simulink model "sampleModel1609"  (R2023a)
settings: Solver=VariableStepAuto  StartTime=0.0  StopTime=10.0  RelTol=1e-3
libraries: hdlsllib x6
settings Model: Creator=user1  LastModifiedBy=user1

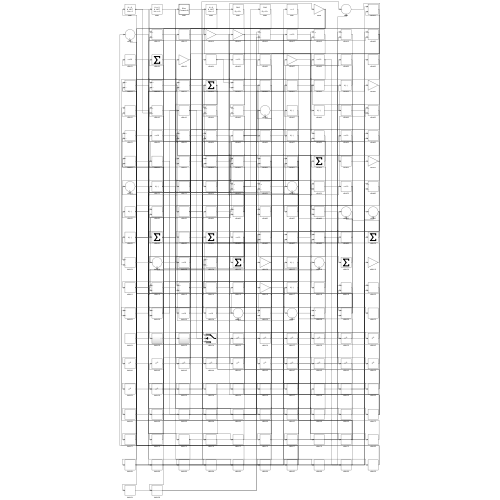
[thumbnail: Simulink's stored preview of the top-level diagram]
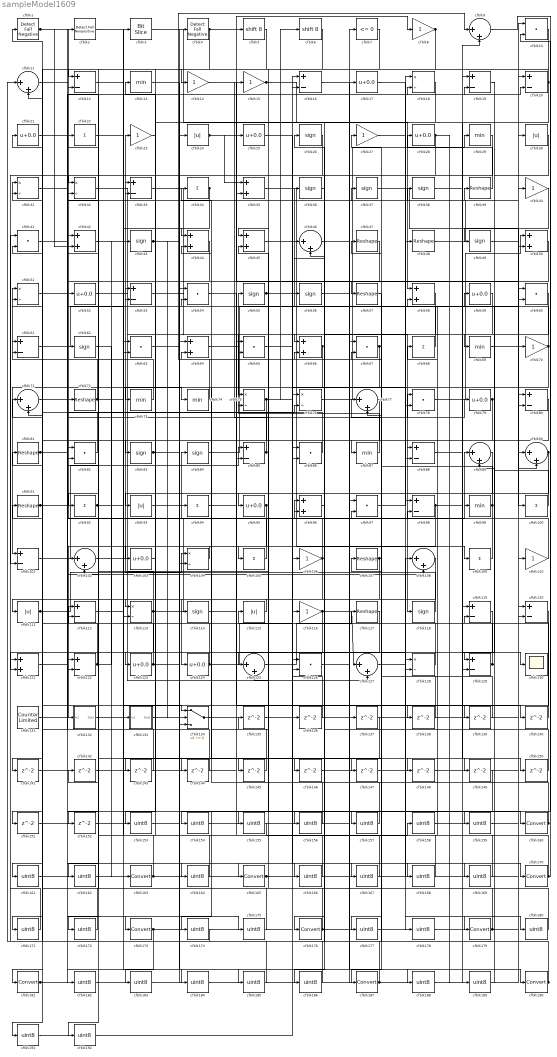
== system sampleModel1609 ==
  cfblk1 : hdlsllib/Logic and Bit Operations/Detect Fall Negative  vinit=0  OutDataTypeStr=boolean
  cfblk{10,41,54,60,63,65,67,78,82,86,97,126} (12 alike) : DotProduct  OutDataTypeStr=Inherit: Inherit via internal rule
  cfblk{22,34,68,92,94,100,105,109} (8 alike) : Sum  Inputs=+
  cfblk{12,16,19..20,33,53,61,80,85,88,98,101,112,119..120,122,129} (17 alike) : Sum  Inputs=+-
  cfblk{9,11,46,71,77,89..90,102,108,125,127} (11 alike) : Sum  Inputs=|++
  cfblk{17,21,25,28,52,59,79,95,103,123..124} (11 alike) : Bias  Bias=0.0  SaturateOnIntegerOverflow=off
  cfblk{18,31..32,51,75..76,104,113,128} (9 alike) : Product  Inputs=*/  RndMeth=Zero  SaturateOnIntegerOverflow=on
  cfblk{8,14..15,23,27,40,70,106,110,116} (10 alike) : Gain
  cfblk{39,47..48,57,72,81,91,107,117} (9 alike) : Reshape
  cfblk{24,30,93,111,115} (5 alike) : Abs  SaturateOnIntegerOverflow=off
  cfblk{26,36..38,43,49,55..56,62,83..84,114,118} (13 alike) : Signum
  cfblk{35,42,44..45,50,58,64,66,96,121} (10 alike) : Sum
  cfblk{13,29,69,73..74,87,99} (7 alike) : MinMax
  cfblk130 : Scope
  cfblk131 : hdlsllib/Sources/Counter Limited  uplimit=7  tsamp=-1
  cfblk132 : Subsystem
      settings: LibrarySourceBlock=|
      | hdlsllib/Ports &
      | Subsystems/Subsystem
  cfblk133 : Subsystem
      settings: LibrarySourceBlock=|
      | hdlsllib/Ports &
      | Subsystems/Subsystem
  cfblk134 : Switch  SaturateOnIntegerOverflow=off  InputSameDT=off
  cfblk{135..152} (18 alike) : Delay  SampleTime=1
  cfblk{153..159,161..162,164,166..169,171..172,174..175,177..178,180,182..186,188..189,191..192} (30 alike) : DataTypeConversion  OutDataTypeStr=uint8  SaturateOnIntegerOverflow=off  RndMeth=Floor
  cfblk{160,163,165,170,173,176,179,181,187,190} (10 alike) : DataTypeConversion  SaturateOnIntegerOverflow=off  RndMeth=Floor
  cfblk2 : hdlsllib/Logic and Bit Operations/Detect Fall Nonpositive  vinit=0  OutDataTypeStr=boolean
  cfblk3 : hdlsllib/Logic and Bit Operations/Bit Slice  lidx=7  ridx=0
  cfblk4 : hdlsllib/Logic and Bit Operations/Detect Fall Negative  vinit=0  OutDataTypeStr=boolean
  cfblk5 : ArithShift  BitShiftNumber=8
  cfblk6 : ArithShift  BitShiftNumber=8
  cfblk7 : hdlsllib/Logic and Bit Operations/Compare To Zero  relop=<=  OutDataTypeStr=boolean
  wires:
  cfblk110/1 -> cfblk89/1
  cfblk15/1 -> cfblk58/1, cfblk105/1
  cfblk105/1 -> cfblk2/1
  cfblk76/1 -> cfblk29/1
  cfblk87/1 -> cfblk55/1
  cfblk74/1 -> cfblk9/1
  cfblk102/1 -> cfblk15/1
  cfblk126/1 -> cfblk160/1
  cfblk104/1 -> cfblk132/1(In1)
  cfblk118/1 -> cfblk23/1
  cfblk116/1 -> cfblk127/1, cfblk192/1
  cfblk35/1 -> cfblk109/1
  cfblk119/1 -> cfblk187/1
  cfblk109/1 -> cfblk84/1
  cfblk82/1 -> cfblk72/1
  cfblk78/1 -> cfblk50/1
  cfblk32/1 -> cfblk127/2
  cfblk84/1 -> cfblk36/1
  cfblk5/1 -> cfblk12/1
  cfblk4/1 -> cfblk83/1, cfblk8/1
  cfblk46/1 -> cfblk17/1
  cfblk62/1 -> cfblk163/1
  cfblk117/1 -> cfblk122/1
  cfblk79/1 -> cfblk118/1, cfblk147/1
  cfblk42/1 -> cfblk75/1
  cfblk73/1 -> cfblk51/1
  cfblk64/1 -> cfblk40/1
  cfblk13/1 -> cfblk165/1
  cfblk97/1 -> cfblk18/1
  cfblk101/1 -> cfblk85/1
  cfblk113/1 -> cfblk99/1, cfblk121/2, cfblk61/2
  cfblk75/1 -> cfblk6/1, cfblk134/3, cfblk138/1
  cfblk83/1 -> cfblk39/1, cfblk20/2
  cfblk81/1 -> cfblk75/2, cfblk33/2
  cfblk25/1 -> cfblk56/1
  cfblk131/1 -> cfblk108/2
  cfblk124/1 -> cfblk1/1, cfblk106/1
  cfblk45/1 -> cfblk70/1
  cfblk41/1 -> cfblk170/1
  cfblk129/1 -> cfblk115/1, cfblk58/2, cfblk89/2
  cfblk12/1 -> cfblk133/1(In1)
  cfblk111/1 -> cfblk104/1, cfblk96/1
  cfblk39/1 -> cfblk28/1
  cfblk107/1 -> cfblk111/1, cfblk125/2
  cfblk80/1 -> cfblk176/1
  cfblk1/1 -> cfblk42/2, cfblk159/1
  cfblk43/1 -> cfblk134/2, cfblk188/1
  cfblk85/1 -> cfblk52/1, cfblk32/2
  cfblk125/1 -> cfblk117/1
  cfblk103/1 -> cfblk53/1
  cfblk106/1 -> cfblk34/1, cfblk152/1
  cfblk134/1 -> cfblk110/1
  cfblk133/1(Out1) -> cfblk94/1
  cfblk52/1 -> cfblk88/1
  cfblk66/1 -> cfblk113/1, cfblk95/1
  cfblk99/1 -> cfblk77/2, cfblk98/2
  cfblk8/1 -> cfblk32/1, cfblk102/1, cfblk171/1
  cfblk34/1 -> cfblk63/2, cfblk44/1
  cfblk123/1 -> cfblk31/1, cfblk78/1
  cfblk98/1 -> cfblk104/2, cfblk150/1
  cfblk11/1 -> cfblk173/1
  cfblk48/1 -> cfblk30/1
  cfblk30/1 -> cfblk49/1
  cfblk44/1 -> cfblk93/1
  cfblk54/1 -> cfblk128/2
  cfblk40/1 -> cfblk69/1
  cfblk67/1 -> cfblk101/1, cfblk144/1, cfblk145/1
  cfblk69/1 -> cfblk90/1
  cfblk14/1 -> cfblk57/1
  cfblk91/1 -> cfblk5/1, cfblk76/2, cfblk79/1
  cfblk49/1 -> cfblk100/1
  cfblk3/1 -> cfblk48/1
  cfblk55/1 -> cfblk116/1, cfblk37/1, cfblk78/2
  cfblk95/1 -> cfblk113/2, cfblk172/1
  cfblk68/1 -> cfblk42/1
  cfblk20/1 -> cfblk14/1, cfblk129/2, cfblk35/2, cfblk46/2
  cfblk58/1 -> cfblk88/2
  cfblk33/1 -> cfblk98/1
  cfblk120/1 -> cfblk181/1
  cfblk57/1 -> cfblk87/1
  cfblk88/1 -> cfblk130/1
  cfblk108/1 -> cfblk124/1
  cfblk96/1 -> cfblk26/1
  cfblk86/1 -> cfblk31/2
  cfblk128/1 -> cfblk81/1
  cfblk114/1 -> cfblk25/1
  cfblk29/1 -> cfblk101/2
  cfblk19/1 -> cfblk129/1
  cfblk70/1 -> cfblk92/1, cfblk12/2
  cfblk100/1 -> cfblk59/1
  cfblk16/1 -> cfblk190/1
  cfblk10/1 -> cfblk45/1
  cfblk28/1 -> cfblk151/1, cfblk189/1
  cfblk122/1 -> cfblk112/1, cfblk102/2, cfblk22/1, cfblk43/1
  cfblk47/1 -> cfblk103/1
  cfblk61/1 -> cfblk3/1
  cfblk37/1 -> cfblk50/2
  cfblk72/1 -> cfblk61/1, cfblk164/1
  cfblk53/1 -> cfblk86/2
  cfblk63/1 -> cfblk66/1
  cfblk21/1 -> cfblk112/2
  cfblk23/1 -> cfblk73/1
  cfblk24/1 -> cfblk18/2, cfblk35/1
  cfblk92/1 -> cfblk38/1, cfblk96/2
  cfblk50/1 -> cfblk122/2
  cfblk121/1 -> cfblk33/1
  cfblk51/1 -> cfblk19/2
  cfblk90/1 -> cfblk123/1, cfblk125/1, cfblk177/1
  cfblk132/1(Out1) -> cfblk134/1
  cfblk27/1 -> cfblk179/1
  cfblk115/1 -> cfblk114/1
  cfblk2/1 -> cfblk74/1
  cfblk136/1 -> cfblk86/1
  cfblk138/1 -> cfblk64/1
  cfblk94/1 -> cfblk139/1
  cfblk139/1 -> cfblk128/1
  cfblk38/1 -> cfblk140/1
  cfblk140/1 -> cfblk53/2
  cfblk26/1 -> cfblk141/1
  cfblk142/1 -> cfblk85/2
  cfblk18/1 -> cfblk143/1
  cfblk143/1 -> cfblk82/1
  cfblk144/1 -> cfblk51/2
  cfblk145/1 -> cfblk54/2
  cfblk89/1 -> cfblk146/1
  cfblk146/1 -> cfblk19/1
  cfblk22/1 -> cfblk148/1
  cfblk148/1 -> cfblk90/2
  cfblk17/1 -> cfblk149/1
  cfblk150/1 -> cfblk66/2
  cfblk151/1 -> cfblk4/1
  cfblk7/1 -> cfblk153/1
  cfblk153/1 -> cfblk24/1
  cfblk9/1 -> cfblk154/1
  cfblk154/1 -> cfblk7/1
  cfblk135/1 -> cfblk155/1
  cfblk59/1 -> cfblk156/1
  cfblk156/1 -> cfblk135/1
  cfblk60/1 -> cfblk157/1
  cfblk157/1 -> cfblk64/2
  cfblk155/1 -> cfblk158/1
  cfblk158/1 -> cfblk60/1
  cfblk159/1 -> cfblk60/2
  cfblk160/1 -> cfblk44/2, cfblk47/1
  cfblk77/1 -> cfblk161/1
  cfblk161/1 -> cfblk126/1
  cfblk137/1 -> cfblk162/1
  cfblk162/1 -> cfblk126/2
  cfblk163/1 -> cfblk76/1, cfblk63/1
  cfblk164/1 -> cfblk62/1
  cfblk165/1 -> cfblk20/1, cfblk108/1
  cfblk152/1 -> cfblk166/1
  cfblk166/1 -> cfblk13/1
  cfblk65/1 -> cfblk167/1
  cfblk167/1 -> cfblk67/1
  cfblk56/1 -> cfblk168/1
  cfblk168/1 -> cfblk65/1
  cfblk93/1 -> cfblk169/1
  cfblk169/1 -> cfblk65/2
  cfblk170/1 -> cfblk10/2, cfblk67/2, cfblk68/1, cfblk77/1
  cfblk171/1 -> cfblk41/1
  cfblk172/1 -> cfblk41/2
  cfblk173/1 -> cfblk136/1, cfblk183/1
  cfblk149/1 -> cfblk174/1
  cfblk174/1 -> cfblk11/1
  cfblk31/1 -> cfblk175/1
  cfblk175/1 -> cfblk11/2
  cfblk176/1 -> cfblk9/2, cfblk82/2
  cfblk177/1 -> cfblk80/1
  cfblk147/1 -> cfblk178/1
  cfblk178/1 -> cfblk80/2
  cfblk179/1 -> cfblk142/1, cfblk97/2, cfblk45/2
  cfblk127/1 -> cfblk180/1
  cfblk180/1 -> cfblk27/1
  cfblk181/1 -> cfblk137/1, cfblk97/1, cfblk54/1
  cfblk141/1 -> cfblk182/1
  cfblk182/1 -> cfblk120/1
  cfblk183/1 -> cfblk120/2
  cfblk71/1 -> cfblk184/1
  cfblk184/1 -> cfblk10/1
  cfblk112/1 -> cfblk185/1
  cfblk185/1 -> cfblk71/1
  cfblk36/1 -> cfblk186/1
  cfblk186/1 -> cfblk71/2
  cfblk187/1 -> cfblk121/1, cfblk46/1, cfblk21/1
  cfblk188/1 -> cfblk119/1
  cfblk189/1 -> cfblk119/2
  cfblk190/1 -> cfblk107/1, cfblk91/1
  cfblk6/1 -> cfblk191/1
  cfblk191/1 -> cfblk16/1
  cfblk192/1 -> cfblk16/2

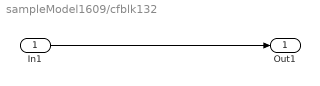
== system sampleModel1609/cfblk132 ==
  In1 : Inport
  Out1 : Outport
  wires:
  In1/1 -> Out1/1

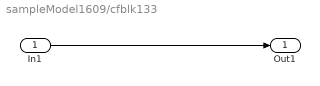
== system sampleModel1609/cfblk133 ==
  In1 : Inport
  Out1 : Outport
  wires:
  In1/1 -> Out1/1
